simulink model "Show_AvoidObstacle_PrintFromOb"  (R2014a)
settings: Solver=FixedStepDiscrete  StartTime=0.0  StopTime=inf  FixedStep=0.033  RelTol=1e-3
libraries: KSim x1
settings Model: Creator=jdelacroix  LastModifiedBy=Bird
settings DataIOCC: SignalLoggingSaveFormat=ModelDataLogs
settings OptimizationCC: ExpressionDepthLimit=2147483647
settings DebuggingCC: UnderspecifiedInitializationDetection=Classic  FcnCallInpInsideContextMsg=EnableAllAsWarning  StateNameClashWarn=warning

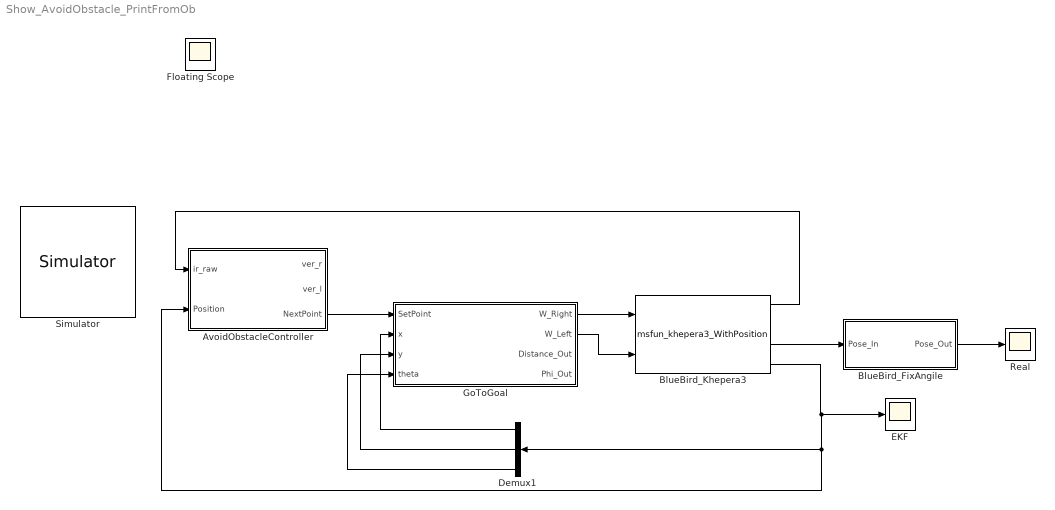
== system Show_AvoidObstacle_PrintFromOb ==
  AvoidObstacleController : MATLAB Function  TreatAsAtomicUnit=on
  BlueBird_FixAngile : MATLAB Function  TreatAsAtomicUnit=on
  BlueBird_Khepera3 : M-S-Function  AncestorBlock=simiam/Khepera III  FunctionName=msfun_khepera3_WithPosition  Parameters=x_0,y_0,theta_0,ShowObservation  mask(Khepera3){x_0=0.4, y_0=0.1, theta_0=0, robot_id=1, ShowObservation=on}
      mask prompts: robot_id "ID"; ShowObservation "显示观测"
      mask Display:
      | port_label('output', 1, 'ir_raw')
      | port_label('output', 2, 'wheel_ticks')
      | port_label('output', 3, 'PosFromSim')
      | port_label('output', 4, 'EKF_Out')
      | 
      | port_label('input', 1, 'vel_r')
      | port_label('input', 2, 'vel_l')
  Demux1 : Demux  Outputs=3
  EKF : Scope
      settings: YMin=-3.5  YMax=3.5  SaveName=ScopeData2
  GoToGoal : MATLAB Function  TreatAsAtomicUnit=on
  Real : Scope
      settings: YMin=-3.5  YMax=3.5
  Simulator : KSim/Simulator  Priority=1
  Floating Scope : Scope
      settings: Floating=on
  wires:
  Demux1/1 -> GoToGoal/2(x)
  Demux1/2 -> GoToGoal/3(y)
  Demux1/3 -> GoToGoal/4(theta)
  AvoidObstacleController/3(NextPoint) -> GoToGoal/1(SetPoint)
  GoToGoal/1(W_Right) -> BlueBird_Khepera3/1
  GoToGoal/2(W_Left) -> BlueBird_Khepera3/2
  BlueBird_Khepera3/1 -> AvoidObstacleController/1(ir_raw)
  BlueBird_Khepera3/4 -> AvoidObstacleController/2(Position), Demux1/1, EKF/1
  BlueBird_Khepera3/3 -> BlueBird_FixAngile/1(Pose_In)
  BlueBird_FixAngile/1(Pose_Out) -> Real/1

== matlab function Show_AvoidObstacle_PrintFromOb/GoToGoal ==
  data: SetPoint input; W_Right output; W_Left output; x input; y input; theta input; Distance_Out output; Phi_Out output
function [W_Right,W_Left,Distance_Out,Phi_Out] = SetPointController(SetPoint,x,y,theta)
%#codegen
goal_x = SetPoint(1,1);
goal_y = SetPoint(2,1);


%系统参数
b = 0.08841;%(m)
r_R = 0.02049915667;%(m)
r_L = 0.02049915667;%(m)
r_Max = max(r_R,r_L);

W_Max = 9.561; %rad/s(43000)
W_Min = (W_Max*2000/43000);%rad/s(2000)

dx = x - goal_x;
dy = y - goal_y;

distance = sqrt(dx * dx + dy * dy);
goalangle = atan2(dy, dx);
%处理一下过大的theta
theta_Use = theta;

Phi = pi + theta_Use - goalangle;

while (Phi > pi) 
    Phi = Phi - 2 * pi;
end

while (Phi < -pi) 
    Phi = Phi + 2 * pi;
end

%开始计算控制器参数
d_1 = 1;%实验平台大小为1m.
K_1 = (r_Max*W_Max)/d_1;
K_1 = K_1 * 4;

d_2 = (W_Min*r_Max)/K_1;
K_3 = W_Min*r_Max;
K_3 = K_3 + 0.0001;

K_2 = K_1*2;

if(distance <= d_2)
    
    %W_Right = (K_1*(distance)*cos(Phi))/r_R - (b*(K_2*Phi + K_1*cos(Phi)*sin(Phi)))/(2*r_R);
    %W_Left = (K_1*(distance)*cos(Phi))/r_L + (b*(K_2*Phi + K_1*cos(Phi)*sin(Phi)))/(2*r_L);
    
    W_Right = (K_3*cos(Phi))/r_R - (b*(K_2*Phi + K_1*cos(Phi)*sin(Phi)))/(2*r_R);
    W_Left = (K_3*cos(Phi))/r_L + (b*(K_2*Phi + K_1*cos(Phi)*sin(Phi)))/(2*r_L);
    
    if(abs(W_Right)<W_Min)
        W_Right = 0;
    end
    if(abs(W_Left)<W_Min)
        W_Left = 0;
    end
    
else
    W_Right = (K_1*(distance)*cos(Phi))/r_R - (b*(K_2*Phi + K_1*cos(Phi)*sin(Phi)))/(2*r_R);
    W_Left = (K_1*(distance)*cos(Phi))/r_L + (b*(K_2*Phi + K_1*cos(Phi)*sin(Phi)))/(2*r_L);
end


Distance_Out = distance;
Phi_Out = Phi;

if(abs(W_Right)>W_Max)
    W_Right = sign(W_Right)*W_Max;
end
if(abs(W_Left)>W_Max)
    W_Left = sign(W_Left)*W_Max;
end

if(distance < 0.01)
    W_Right = 0;
    W_Left = 0;
end

== matlab function Show_AvoidObstacle_PrintFromOb/AvoidObstacleController ==
  data: ir_raw input; ver_r output; ver_l output; Position input; NextPoint output
function [ver_r,ver_l,NextPoint] = AvoidObstacle(ir_raw,Position)
%#codegen

%没有噪声的前提下，将原始红外数据转换为距离
ir_distances = IR_Raw_to_Distances(ir_raw);
%由于红外传感器在x正轴方向安装的比负方向多，将传感器9的数值+一点，加以修正

FixIR_9_Number = 0.364;%应该补偿0.3642，现在少补偿一点，让平时，机器人的向量决策为当前机器人的前方
ir_distances = ir_distances + ([0 0 0 0 0 0 0 0 1]')*FixIR_9_Number;
%利用红外距离数据计算以机器人坐标的周围物体：
Obstacle_AroundRobot = zeros(3,9);
for i = 1:1:9%一共有九个红外
     IR_Position_I = GetIR_Position(i);
     IR_Transformation_Matrix_I = Transformation_Matrix(IR_Position_I(1,1),IR_Position_I(2,1),IR_Position_I(3,1));
     Obstacle_AroundRobot_I = IR_Transformation_Matrix_I*[ir_distances(i) ; 0 ; 1];
     
     Obstacle_AroundRobot(:,i) = Obstacle_AroundRobot_I;
end
%将以机器人为原点的周围障碍物信息转换为以世界坐标系的信息
Obstacle_AroundRobot_World = Transformation_Matrix(Position(1,1), Position(2,1), Position(3,1))*Obstacle_AroundRobot;

%进入控制器
%[v,w] = AvoidObstacles_GeorgiaInstitute(Obstacle_AroundRobot_World,Position);
NextPoint = AvoidObstacles_NextPoint(Obstacle_AroundRobot_World,Position);

%[ver_r, ver_l] = diff_to_uni(v,w);
ver_r = 1;
ver_l = 1;
end

%% 下面是帮助函数库
function [Answer] = Transformation_Matrix(x, y, theta)
    %坐标转移矩阵
    AvoidObstacles_Use = simiam.controller.AvoidObstacles();
    Answer = AvoidObstacles_Use.get_transformation_matrix(x, y, theta);
end

function [Answer] = IR_Raw_to_Distances(ir_raw)
    %将传感器数据转换为距离
    %reallog就是以e为底的对数
    SafeNumber = 150;
    MaxNumber = 3960;
    
    ir_raw_Internal = ir_raw;
    
    %处理掉ir_raw_Internal里面<SafeNumber的数值
    Number_List = find(ir_raw_Internal < SafeNumber);
    ir_raw_Internal(Number_List) = SafeNumber;
    
    %处理掉超过允许最大值的值
    Number_List = find(ir_raw_Internal > MaxNumber);
    ir_raw_Internal(Number_List) = MaxNumber;
    
    Answer = 0.02-reallog(ir_raw_Internal/3960)/30;
end

function [Answer] = GetIR_Position(IR_Number)
    Pose2D_Use = simiam.ui.Pose2D(0,0,0);
    IR_Position = [
        -0.038  0.049 Pose2D_Use.deg2rad(128);
        0.017  0.063  Pose2D_Use.deg2rad(75);
        0.051  0.045  Pose2D_Use.deg2rad(42);
        0.067  0.015  Pose2D_Use.deg2rad(13);
        0.067  -0.015  Pose2D_Use.deg2rad(-13);
        0.051  -0.045  Pose2D_Use.deg2rad(-42);
        0.017  -0.063  Pose2D_Use.deg2rad(-75);
        -0.038  -0.049  Pose2D_Use.deg2rad(-128);
        -0.052  0.000  Pose2D_Use.deg2rad(180)
    ];
    Answer = (IR_Position(IR_Number,:))';
    %Answer = 0;
end

function [r,l] = diff_to_uni(v,w)
    R = 0.02049915667;
    L = 0.08841;

    r = v/R + (w*L)/(2*R);
    l = v/R - (w*L)/(2*R);
end

function [v,w] = AvoidObstacles_GeorgiaInstitute(Obstacle_AroundRobot_World,Position)
%http://www.gatech.edu/welcome
%乔治理工的控制器
persistent Last_e_P Last_e_I
if isempty(Last_e_P)
    Last_e_P = 0;
    Last_e_I = 0;
end

%障碍物坐标向量权重
sensor_gains = [1 1 1 1 1 1 1 1 1];

Kp = 5;
Ki = 0;
Kd = 0;

%(ir_distances_rf-repmat([x;y],1,9))这个是以机器人为起点，以障碍物为终点的向量列
%去掉Obstacle_AroundRobot_World里面的最后一行1
ir_distances_rf = Obstacle_AroundRobot_World(1:2,:);
u_i = (ir_distances_rf-repmat([Position(1,1);Position(2,1)],1,9))*diag(sensor_gains);
%u_i是给每一个障碍物向量加一个权重，正如说明书上写的
%然后把这些向量加起来,得到最不可能有障碍物方向的向量
u_ao = sum(u_i,2);

% Compute the heading and error for the PID controller
theta_o = atan2(u_ao(2),u_ao(1));%向量的方向角
e_k = theta_o-Position(3);%方向角误差
e_k = atan2(sin(e_k),cos(e_k));

dt = 0.033;
%只对方向角误差进行修正
e_P = e_k;
%e_I = 0;
%e_D = 0;
e_I = Last_e_I + e_P*dt;
e_D = (e_P-Last_e_P)/dt;

%保存以备下一次使用：
Last_e_P = e_P;
Last_e_I = e_I;
    
w = Kp*e_P + Ki*e_I + Kd*e_D;
v =  0.25/(log(abs(w)+2)+1);
end

function [NextPoint] = AvoidObstacles_NextPoint(Obstacle_AroundRobot_World,Position)
FixIR_9_Number = 0.364;

%障碍物坐标向量权重
sensor_gains = [1 1 1 1 1 1 1 1 1];
%(ir_distances_rf-repmat([x;y],1,9))这个是以机器人为起点，以障碍物为终点的向量列
%去掉Obstacle_AroundRobot_World里面的最后一行1
ir_distances_rf = Obstacle_AroundRobot_World(1:2,:);
u_i = (ir_distances_rf-repmat([Position(1,1);Position(2,1)],1,9))*diag(sensor_gains);
%u_i是给每一个障碍物向量加一个权重，正如说明书上写的
%然后把这些向量加起来,得到最不可能有障碍物方向的向量
SumOfObstacleVector_Word = sum(u_i,2);
NextAngle = atan2(SumOfObstacleVector_Word(2,1),SumOfObstacleVector_Word(1,1));

%找到周围最远的障碍物，就是最空旷的地方
d_List = sqrt(u_i(1,:).^2 + u_i(2,:).^2);
d_List(9) = d_List(9) - FixIR_9_Number;%应该补偿0.3642，现在少补偿一点，让平时，机器人的向量决策为当前机器人的前方
d_List = max(d_List);
d_List = d_List - 0.07;%减去的是机器人的半径
if(d_List < 0)
    d_List = 0.001;%如果障碍物都很近，则设置一个在停止距离以内的点，机器人认为到了这个点，就停止下来不走了
end

%下面计算下一个点的坐标，用圆的参数方程
NextPoint_X = Position(1,1) + d_List*cos(NextAngle);
NextPoint_Y = Position(2,1) + d_List*sin(NextAngle);
NextPoint = [NextPoint_X ; NextPoint_Y];
%Temp = 0;
end

== matlab function Show_AvoidObstacle_PrintFromOb/BlueBird_FixAngile ==
  data: Pose_Out output; Pose_In input
function Pose_Out = FixAngile(Pose_In)
%用来修正过大的角度，输入域是：-pi-pi
Rad = Pose_In(3,1);
while (Rad > pi) 
    Rad = Rad - 2 * pi;
end
while (Rad < -pi) 
    Rad = Rad + 2 * pi;
end

Pose_Out = Pose_In;
Pose_Out(3,1) = Rad;
